simulink model "proj"  (R2016a)
settings: Solver=FixedStepAuto  StartTime=0.0  StopTime=.5  RelTol=1e-3
libraries: dspsrcs4 x5, commanabbnd3 x2, dspfdesign x2, dspvision x1
settings Model: Creator=swhuber  LastModifiedBy=swhuber

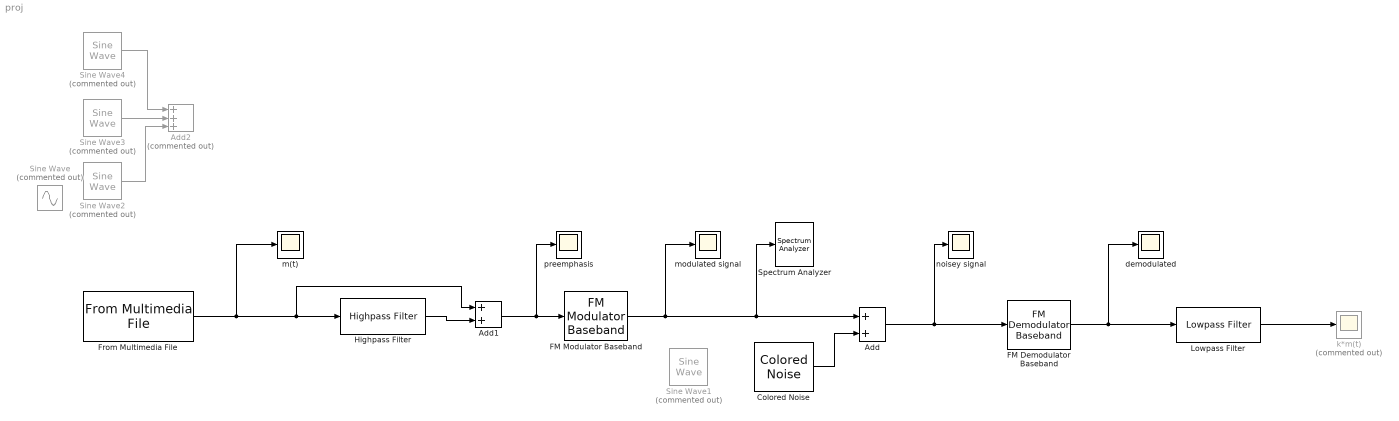
== system proj ==
  Add : Sum  LockScale=on
  Add1 : Sum
  Add2 : Sum  Commented=on  Inputs=+++
  Colored Noise : dspsrcs4/Colored Noise  Color=purple  InverseFrequencyPower=1  NumChannels=1  OutputDataType=double  SamplesPerFrame=1024  SampleTime=1  RandomStream=mt19937ar with seed  Seed=67  SimulateUsing=Interpreted execution
  "FM Demodulator Baseband " : commanabbnd3/FM Demodulator Baseband   FrequencyDeviation=75e3  SimulateUsing=Code generation
  FM Modulator Baseband : commanabbnd3/FM Modulator Baseband  FrequencyDeviation=75e3  SimulateUsing=Code generation
  From Multimedia File : dspvision/From Multimedia File  inputFilename=\\my.files.iastate.edu\Users\swhuber\Desktop\ass.mp3  loop=on  numPlays=1  outputStreams=Audio only  videoDataType=single  audioDataType=double  inheritSampleTime=on  userDefinedSampleTime=1/30  noAudioOutput=off  isIntensityVideo=off  fourcc=RGB  colorVideoFormat=Separate color signals  outputEOF=off  dataOrg=Column-major  audioFrameSize=1024  computeAudioFrameSize=off  outSamplingMode=Sample based
  Highpass Filter : dspfdesign/Highpass Filter  FilterType=IIR  DesignForMinimumOrder=on  FilterOrder=50  StopbandFrequency=1000  PassbandFrequency=1200  StopbandAttenuation=60  PassbandRipple=.1  InheritSampleRate=off  SampleRate=44100  roundingMode=Floor  coeffsDataTypeStr=fixdt(1,16)  SimulateUsing=Interpreted execution
  Lowpass Filter : dspfdesign/Lowpass Filter  FilterType=FIR  DesignForMinimumOrder=on  FilterOrder=50  PassbandFrequency=8e3  StopbandFrequency=12e3  PassbandRipple=0.1  StopbandAttenuation=80  InheritSampleRate=off  SampleRate=44100  roundingMode=Floor  coeffsDataTypeStr=fixdt(1,16)  SimulateUsing=Interpreted execution
  Sine Wave : Sin  Commented=on  SineType=Sample based  Amplitude=5  Frequency=3000*pi  Samples=1000  SampleTime=.0000006666
  Sine Wave1 : dspsrcs4/Sine Wave  Commented=on  Amplitude=1  Frequency=100  Phase=0  SampleMode=Discrete  OutComplex=Real  CompMethod=Trigonometric fcn  TableSize=Speed  SampleTime=1/1500000  SamplesPerFrame=1  ResetState=Restart at time zero  OutputFrames=off  dataType=double  wordLen=16  udDataType=sfix(16)  fracBitsMode=Best precision  numFracBits=15  OutDataTypeStr=double  LastOutDataTypeStr=double
  Sine Wave2 : dspsrcs4/Sine Wave  Commented=on  Amplitude=1  Frequency=1500  Phase=0  SampleMode=Discrete  OutComplex=Real  CompMethod=Trigonometric fcn  TableSize=Speed  SampleTime=1/1500000  SamplesPerFrame=1  ResetState=Restart at time zero  OutputFrames=off  dataType=double  wordLen=16  udDataType=sfix(16)  fracBitsMode=Best precision  numFracBits=15  OutDataTypeStr=double  LastOutDataTypeStr=double
  Sine Wave3 : dspsrcs4/Sine Wave  Commented=on  Amplitude=1  Frequency=100  Phase=pi/2  SampleMode=Discrete  OutComplex=Real  CompMethod=Trigonometric fcn  TableSize=Speed  SampleTime=1/1500000  SamplesPerFrame=1  ResetState=Restart at time zero  OutputFrames=off  dataType=double  wordLen=16  udDataType=sfix(16)  fracBitsMode=Best precision  numFracBits=15  OutDataTypeStr=double  LastOutDataTypeStr=double
  Sine Wave4 : dspsrcs4/Sine Wave  Commented=on  Amplitude=1  Frequency=2000  Phase=pi  SampleMode=Discrete  OutComplex=Real  CompMethod=Trigonometric fcn  TableSize=Speed  SampleTime=1/1500000  SamplesPerFrame=1  ResetState=Restart at time zero  OutputFrames=off  dataType=double  wordLen=16  udDataType=sfix(16)  fracBitsMode=Best precision  numFracBits=15  OutDataTypeStr=double  LastOutDataTypeStr=double
  Spectrum Analyzer : SpectrumAnalyzer
  demodulated : Scope
  k*m(t) : Scope  Commented=on
  m(t) : Scope
  modulated signal : Scope
  noisey signal : Scope
  preemphasis : Scope
  wires:
  Add1/1 -> FM Modulator Baseband/1, preemphasis/1
  Add/1 -> "FM Demodulator Baseband "/1, noisey signal/1
  "FM Demodulator Baseband "/1 -> demodulated/1, Lowpass Filter/1
  Lowpass Filter/1 -> k*m(t)/1
  Colored Noise/1 -> Add/2
  Highpass Filter/1 -> Add1/2
  From Multimedia File/1 -> Add1/1, Highpass Filter/1, m(t)/1
  Sine Wave4/1 -> Add2/1
  Sine Wave3/1 -> Add2/2
  Sine Wave2/1 -> Add2/3
  FM Modulator Baseband/1 -> Spectrum Analyzer/1, Add/1, modulated signal/1
